simulink model "SolutionP145"  (Simulink 9.2)
settings: Solver=VariableStepAuto  StartTime=0.0  StopTime=tmax  MaxStep=0.1  RelTol=1e-3
values from neighbouring files (symbols this model uses):
  a0 = 1    [SolutionP1.m]    (also in SolutionP22.m; SolutionP31.m)
  a1 = 0.5    [SolutionP1.m]    (also in SolutionP22.m = 0.2; SolutionP2KalmanFilter.m = -1.5; SolutionP31.m = 0.2)
  b0 = 1    [SolutionP1.m]    (also in SolutionP22.m; SolutionP2KalmanFilter.m = 0.9; SolutionP31.m)
settings Model: Creator=raphael  LastModifiedBy=raphael
settings DataIOCC: LimitDataPoints=off  SaveFormat=Dataset  SignalLoggingSaveFormat=Dataset
settings OptimizationCC: LifeSpan=auto
settings DebuggingCC: UnderspecifiedInitializationDetection=Simplified  MergeDetectMultiDrivingBlocksExec=error  FcnCallInpInsideContextMsg=error  StateNameClashWarn=none  SFUnexpectedBacktrackingDiag=error  SFNoUnconditionalDefaultTransitionDiag=error  SFExecutionAtInitializationDiag=warning
settings HardwareCC: ProdBitPerPointer=64  ProdBitPerSizeT=64  ProdBitPerPtrDiffT=64  ProdLargestAtomicFloat=Float  ProdIntDivRoundTo=Zero  ProdEndianess=LittleEndian  ProdWordSize=64  ProdHWDeviceType=Intel->x86-64 (Windows64)
settings ModelReferenceCC: PropagateSignalLabelsOutOfModel=on
settings SFSimCC: SimUseLocalCustomCode=on
settings RTWCC: RTWUseLocalCustomCode=on
settings CodeAppCC: StateflowObjectComments=off
settings GRTTargetCC: TargetLangStandard=C99 (ISO)  GeneratePreprocessorConditionals=Use local settings  CombineOutputUpdateFcns=on  GRTInterface=off
settings ConfigComp: CovMetricSettings=dwe  CovHtmlReporting=off  CovSaveCumulativeToWorkspaceVar=off  CovSaveSingleToWorkspaceVar=off  CovExternalEMLEnable=on

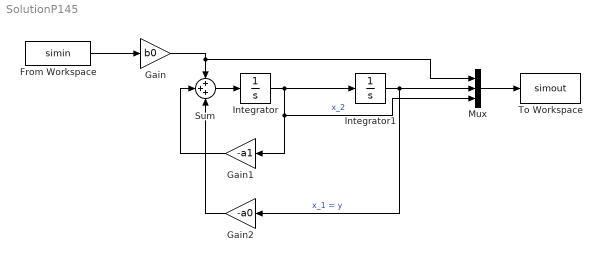
== system SolutionP145 ==
  From Workspace : FromWorkspace  VariableName=simin  SampleTime=0
  Gain : Gain  Gain=b0
  Gain1 : Gain  Gain=-a1
  Gain2 : Gain  Gain=-a0
  Integrator : Integrator
  Integrator1 : Integrator
  Mux : Mux  Inputs=3
  Sum : Sum  Inputs=+++
  To Workspace : ToWorkspace  VariableName=simout  SaveFormat=Timeseries  SampleTime=-1
  wires:
  Sum/1 -> Integrator/1
  Integrator/1 -> Integrator1/1, Mux/3, Gain1/1  "x_2"
  Gain1/1 -> Sum/2
  Gain/1 -> Mux/1, Sum/1
  From Workspace/1 -> Gain/1
  Integrator1/1 -> Gain2/1, Mux/2  "x_1 = y"
  Gain2/1 -> Sum/3
  Mux/1 -> To Workspace/1
